simulink model "sm_excv_track1_float"  (R2026a)
settings: Solver=ode23t  StopTime=20  FixedStep=2e-4  AbsTol=1e-3
StartFcn:
  | tic
StopFcn:
  | Elapsed_Sim_Time = toc;
  | disp(['Elapsed Sim Time = ' num2str(Elapsed_Sim_Time)]);
undefined symbols (not defined in the file or in its folder): Excv
libraries: sm_lib x3, fl_lib x2, nesl_utility x2, sm_excv_chassis_lib x1, sm_trackV_lib_chain_underc_elem x1, simulink x1, sm_trackV_lib_chain_lower_frame_s46i1u2l7 x1
CloseFcn:
  | try,close(h1_sm_excv_track_single_float),end
  | clear h1_sm_excv_track_single_float
  | try,close(h2_sm_excv_track_single_float),end
  | clear h2_sm_excv_track_single_float
  | try,close(h3_sm_excv_track_single_float),end
  | clear h3_sm_excv_track_single_float
  | try,close(h4_sm_excv_track_single_float),end
  | clear h4_sm_excv_track_single_float
  | 
  | 
  | clear simlog_sm_excv_track_single_float
  | clear logsout_sm_excv_track_single_float
Description:
  | Excavator Track (Single) Suspended in Air
  | Copyright 2023-2026 The MathWorks, Inc.
settings Model: Creator=evo  LastModifiedBy=smiller
settings SolverCC: ExtrapolationOrder=1.0
settings DataIOCC: SignalLoggingName=logsout_sm_excv_track1_float
settings DebuggingCC: SymbolicDimsDataTypeCodeGenerationDiagnostic=none
settings SimscapeCC: SimscapeNominalValues="[{\"value\":\"1\",\"unit\":\"A\"},{\"value\":\"1\",\"unit\":\"bar\"},{\"value\":\"1\",\"unit\":\"cm^2\"},{\"value\":\"1\",\"unit\":\"cm^3/s\"},{\"value\":\"1\",\"unit\":\"kJ/kg\"},{\"value\":\"1\",\"unit\":\"kW\"},{\"value\":\"1\",\"unit\":\"l\"},{\"value\":\"1\",\"unit\":\"N\"},{\"value\":\"1\",\"unit\":\"N*m\"},{\"value\":\"1\",\"unit\":\"V\"}]"  SimscapeLogSimulationStatistics=on  SimscapeLogName=simlog_sm_excv_track1_float  SimscapeLogLimitData=off
settings DiagnosticsConfigSet: SimMechanicsConflictingReferenceFrames=none
settings ExplorerConfigSet: InternalSimMechanicsExplorerSettings="<ExplorerConfiguration><canonicalview>default</canonicalview><AnimationSetting><BasePlaybackSpeed>1.0</BasePlaybackSpeed><PlaybackSpeedFactor>1.0</PlaybackSpeedFactor></AnimationSetting><TilePanel><TileInfo><Tiles Columns=\"1\" Count=\"1\" Rows=\"1\"><Column Weight=\"1\"/><Row Weight=\"1\"/><Tile Height=\"1\" Width=\"1\" X=\"0\" Y=\"0\"/></Tiles></TileInfo><SceneInfo><SceneViewer><BGColor><R>1</R><G>1</G><B>1</B></BGColor><Camera><DoPerspective>off</DoPerspective><Position><X>1.74609408504787811</X><Y>-1.4110954799022255</Y><Z>0.03793465708004784</Z></Position><Center><X>1.74609408504787811</X><Y>1.1000000413852602</Y><Z>0.03793465708004784</Z></Center><Up><X>0</X><Y>-0</Y><Z>1</Z></Up><ViewLimDist>1</ViewLimDist><YLim>1.28209836141025391</YLim><XLim>2.245186421871185</XLim></Camera></SceneViewer></SceneInfo></TilePanel><MechEditorPanel><Cameras/><GfxPanelCameraMap/><VideoCreator><PlaybackSpeedRatio>1.0</PlaybackSpeedRatio><FrameRate>30</FrameRate><VideoFormat>Motion JPEG AVI</VideoFormat><FrameSize>auto</FrameSize></VideoCreator></MechEditorPanel></ExplorerConfiguration>"

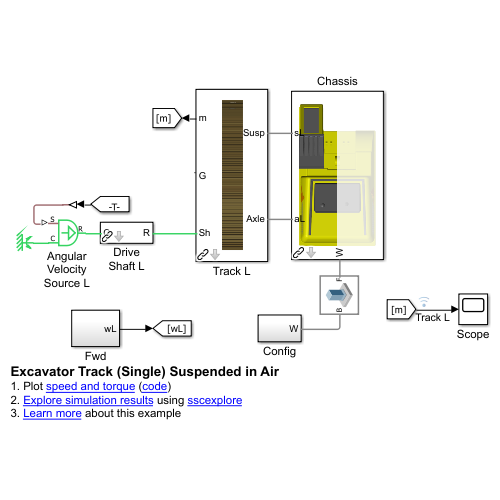
[thumbnail: Simulink's stored preview of the top-level diagram]
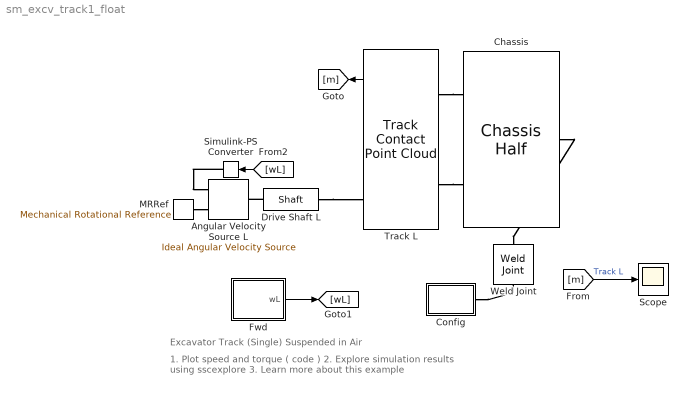
== system sm_excv_track1_float ==
  note: Excavator Track (Single) Suspended in Air
  note: 1. Plot speed and torque ( code )
      | 2. Explore simulation results using sscexplore
      | 3. Learn more about this example
  Angular Velocity Source L : fl_lib/Mechanical/Mechanical Sources/Ideal Angular Velocity Source
  Chassis : sm_excv_chassis_lib/Chassis Half  Camera=Excv.Chassis.Camera  offset_cg=Excv.Chassis.CGOffset  offset_axle=Excv.Chassis.AxleOffset  offset_sprk2axle_x=Excv.Frame.AxleX  offset_sprk2axle_y=Excv.Frame.AxleY  track_sep_ctr=Excv.Chassis.TrackSepCtr  chassis_mass=Excv.Chassis.Mass/2  chassis_moi=Excv.Chassis.MOI/2  chassis_poi=Excv.Chassis.POI/2
  Config : Subsystem
  Drive Shaft L : sm_trackV_lib_chain_underc_elem/Shaft  k_shaft=Excv.Drive.Shaft.k  b_shaft=Excv.Drive.Shaft.b
  Fwd : Subsystem  VariantControl=Fwd
  MRRef : fl_lib/Mechanical/Rotational Elements/Mechanical Rotational Reference
  Scope : Scope
      settings: ActiveDisplayYMinimum=-11747.25975  ActiveDisplayYMaximum=35828.2276
  Simulink-PS Converter : nesl_utility/Simulink-PS Converter  PhysicalDomain=network_engine_domain  SubClassName=ps_input  LeftPortType=input  RightPortType=output  PseudoPeriodic=off  Frequencies=[]  NoiseDistribution=none  NoiseParameters=[]  Unit=1  AffineConversion=off  FilteringAndDerivatives=provide  SimscapeFilterOrder=1  InputFilterTimeConstant=0.001  UdotUserProvided=0
  Track L : sm_trackV_lib_chain_lower_frame_s46i1u2l7/Track Contact Point Cloud  popup_leftOrRight=Left  sprk_xc=Excv.Sprocket.sprocket_xc  sprk_len=Excv.Sprocket.sprk_width  sprk_rho=Excv.Sprocket.density  sprk_clr=Excv.Sprocket.clr  sprk_opc=Excv.Sprocket.opc  sprk_contact_geo_ptcld=Excv.Sprocket.teeth_contact.ptcld.pts  sprk_contact_geo_rad=Excv.Sprocket.teeth_contact.ptcld.rad  sprk_contact_geo_clr=Excv.Sprocket.teeth_contact.ptcld.clr  sprk_contact_geo_opc=Excv.Sprocket.teeth_contact.ptcld.opc  idler_rad=Excv.Idler.rad  idler_len=Excv.Idler.len  idler_rho=Excv.Idler.rho  idler_clr=Excv.Idler.clr  idler_opc=Excv.Idler.opc  idler_contgeo_clr=Excv.Idler.chain_contact.clr  idler_contgeo_opc=Excv.Idler.chain_contact.opc  roller_upper_rad=Excv.Roller.Upper.rad  roller_upper_len=Excv.Roller.Upper.len  roller_upper_rho=Excv.Roller.Upper.rho  roller_upper_clr=Excv.Roller.Upper.clr  roller_upper_opc=Excv.Roller.Upper.opc  roller_upper_contgeo_clr=[1.0 0.0 0.0]  roller_upper_contgeo_opc=1  roller_lower_rad=Excv.Roller.Lower.rad  roller_lower_len=Excv.Roller.Lower.len  roller_lower_rho=Excv.Roller.Lower.rho  roller_lower_clr=Excv.Roller.Lower.clr  roller_lower_opc=Excv.Roller.Lower.opc  roller_lower_contgeo_clr=[1.0 0.0 0.0]  roller_lower_contgeo_opc=1  tensioner_cyl_len=Excv.Idler.Tensioner.cyl.len  tensioner_cyl_rad=Excv.Idler.Tensioner.cyl.rad  tensioner_cyl_rho=Excv.Idler.Tensioner.cyl.rho  tensioner_cyl_clr=Excv.Idler.Tensioner.cyl.clr  tensioner_cyl_opc=Excv.Idler.Tensioner.cyl.opc  tensioner_pist_len=Excv.Idler.Tensioner.piston.len  tensioner_pist_rad=Excv.Idler.Tensioner.piston.rad  tensioner_pist_rho=Excv.Idler.Tensioner.piston.rho  tensioner_pist_clr=Excv.Idler.Tensioner.piston.clr  tensioner_pist_opc=Excv.Idler.Tensioner.piston.opc  tensioner_br_length=Excv.Idler.Tensioner.bracket.len  tensioner_br_width=Excv.Idler.Tensioner.bracket.wid  tensioner_br_height=Excv.Idler.Tensioner.bracket.height  tensioner_br_thk=Excv.Idler.Tensioner.bracket.thk  tensioner_br_rho=Excv.Idler.Tensioner.bracket.rho  tensioner_br_clr=Excv.Idler.Tensioner.bracket.clr  tensioner_br_opc=Excv.Idler.Tensioner.bracket.opc  tensioner_eqpos=Excv.Idler.Tensioner.xeq  tensioner_x0=Excv.Idler.Tensioner.x0  tensioner_k=Excv.Idler.Tensioner.K  tensioner_b=Excv.Idler.Tensioner.B  roller_upper_x=Excv.Frame.Sprk2UpperX  roller_lower_x=Excv.Frame.Sprk2LowerX  idler_x=Excv.Frame.IdlerAssyX  axle_x=Excv.Frame.AxleX  roller_upper_y=Excv.Frame.Sprk2UpperY  roller_lower_y=Excv.Frame.Sprk2LowerY  idler_y=Excv.Frame.Sprk2IdlerY  sprk_pitch_rad=Excv.Sprocket.sprocket_rPitch  axle_y=Excv.Frame.AxleY  frame_cg_offset=Excv.Frame.CGOffset  frame_mass=Excv.Frame.Mass  frame_moi=Excv.Frame.MOI  frame_poi=Excv.Frame.POI  frame_susp_offset=Excv.Frame.SuspOffset  chain_wid=Excv.Chain.chain_wid  chain_seg_m=Excv.Chain.link_m  chain_seg_cg=Excv.Chain.link_cg  chain_seg_moi=Excv.Chain.link_moi  chain_seg_poi=Excv.Chain.link_poi  plate_xc=Excv.Chain.plate_xc  plate_h=Excv.Chain.plate_h  pin_sep=Excv.Chain.pin_sep  plate_thk=Excv.Chain.plate_thk  plate_ang=Excv.Chain.plate_ang  plate_clr=Excv.Chain.plate_clr  plate_opc=Excv.Chain.plate_opc  pin_len=Excv.Chain.pin_len  pin_rad=Excv.Chain.pin_rad  pin_clr=Excv.Chain.pin_clr  pin_opc=Excv.Chain.pin_opc  shoe_xc=Excv.Shoe.xc  shoe_w=Excv.Shoe.w  shoe_m=Excv.Shoe.mass  shoe_cg=Excv.Shoe.cg  shoe_moi=Excv.Shoe.moi  shoe_poi=Excv.Shoe.poi  shoe_clr=Excv.Shoe.clr  shoe_opc=Excv.Shoe.opc  jointTargets=track_joint_targets  chainDamping=Excv.Chain.damping  ptcld_shoe=Excv.Shoe.ground_contact.ptcld.pts  ptcld_shoe_rad=Excv.Shoe.ground_contact.ptcld.rad  ptcld_shoe_clr=Excv.Shoe.ground_contact.ptcld.clr  ptcld_shoe_opc=Excv.Shoe.ground_contact.ptcld.opc  chain_to_roller_clr=Excv.Chain.roller_contact.clr  chain_to_roller_opc=Excv.Chain.roller_contact.opc  chain_to_teeth_clr=Excv.Chain.teeth_contact.clr  chain_to_teeth_opc=Excv.Chain.teeth_contact.opc  B_Sprocket=Excv.Contact.Sprocket.B  K_Sprocket=Excv.Contact.Sprocket.K  TW_Sprocket=Excv.Contact.Sprocket.TW  K_Roller=Excv.Contact.Roller.K  B_Roller=Excv.Contact.Roller.B  TW_Roller=Excv.Contact.Roller.TW  K_Idler=Excv.Contact.Idler.K  B_Idler=Excv.Contact.Idler.B  TW_Idler=Excv.Contact.Idler.TW  popup_sense_roller=Actuator Torque
  Weld Joint : sm_lib/Joints/Weld Joint  JointMode=Normal  CompositeWrenchDir=FollowerOnBase  CompositeWrenchFrame=BaseFrame  SenseConstraintForce=off  SenseConstraintTorque=off  SenseTotalForce=off  SenseTotalTorque=off
  wires:
  Track L/1 -> [m]
  [m] -> Scope/1  "Track L"
  [wL] -> Simulink-PS Converter/1
  Fwd/1(wL) -> [wL]
  connections:
  Config/LConn1 -- Weld Joint/LConn1
  Chassis/RConn1 -- Weld Joint/RConn1
  Simulink-PS Converter/RConn1 -- Angular Velocity Source L/RConn1
  MRRef/LConn1 -- Angular Velocity Source L/RConn2
  Drive Shaft L/LConn1 -- Angular Velocity Source L/LConn1
  Track L/LConn1 -- Chassis/LConn1
  Track L/LConn2 -- Chassis/LConn2
  Drive Shaft L/RConn1 -- Track L/RConn2

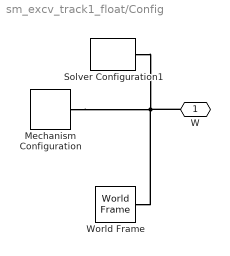
== system sm_excv_track1_float/Config ==
  Mechanism Configuration : sm_lib/Utilities/Mechanism Configuration  UniformGravity=Constant  GravityVector=[-9.80665 0 0]  GravityVectorUnits=m/s^2  LinearizationDelta=0.001  JointModeTransitionNonlinearIterations=2
      settings: AttributesFormatString=Gravity: %<GravityVector>
  Solver Configuration1 : nesl_utility/Solver Configuration  PhysicalDomain=network_engine_domain  SubClassName=solver  LeftPortType=input  RightPortType=generic  Tones=[]  Harmonics=[]  SimulateNoise=off  Profile=off  UseLocalSampling=off  EnableSwitchedLinearOptims=on  FrequencyDomain=off  UseCCode=off  RelTol=0.001  AbsTol=0.001  MinStep=1e-09  ToWorkspace=off  RevertToSquareIcSolve=off  NumHomotopyIterations=100  PhasorMode=off  PhasorModeNumHarmonics=1  ConsistencySolver=NEWTON_FTOL  CanonicalOrdering=UNORDERED  OptimizeIntermediates=UNOPTIMIZED  IndexReductionMethod=DerivativeReplacement  DoDC=off  ResidualTolerance=1e-09  ConsistencyTolSource=GLOBAL  ConsistencyAbsTol=0.001  ConsistencyRelTol=0.001  ConsistencyTolFactor=0.001  UseLocalSolver=off  LocalSolverChoice=NE_BACKWARD_EULER_ADVANCER  ResolveIndetEquations=on  FunctionEvalNumThread=1  LocalSolverSampleTime=0.001  DoFixedCost=off  MaxNonlinIter=3  MaxModeIter=2  ComputeImpulses=off  ImpulseIterations=2  LinearAlgebra=auto  LinearAlgebraNumThread=0  EquationFormulation=NE_TIME_EF  DelaysMemoryBudget=1024  AutomaticFiltering=on  FilteringTimeConstant=0.001  PartitionStorageMethod=AS_NEEDED  PartitionMemoryBudget=1024  PartitionMethod=ROBUST  MultibodyUseLocalSolver=off  MultibodyLocalSolverChoice=ODE1  MultibodyLocalSolverSampleTime=0.001
  World Frame : sm_lib/Frames and Transforms/World Frame
  W : PMIOPort  Side=Left
  connections:
  W/RConn1 -- Solver Configuration1/RConn1 -- Mechanism Configuration/RConn1 -- World Frame/RConn1

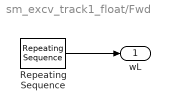
== system sm_excv_track1_float/Fwd ==
  Repeating Sequence : simulink/Sources/Repeating Sequence  rep_seq_t=[0 2 2.01 40]  rep_seq_y=[0 0 3 3]
  wL : Outport
  wires:
  Repeating Sequence/1 -> wL/1
